simulink model "Simulink_disco"  (R2024a)
settings: Solver=VariableStepAuto  StartTime=0.0  StopTime=10.0  RelTol=1e-3
values from neighbouring files (symbols this model uses):
  k = 100    [Ec3.m]    (also in Simulink_datos.m)
  m = 10    [Ec3.m]    (also in Simulink_datos.m)
  r = 0.05    [Ec3.m]    (also in Simulink_datos.m)
settings Model: Creator=Braulio Ramíreza  LastModifiedBy=Braulio Ramíreza

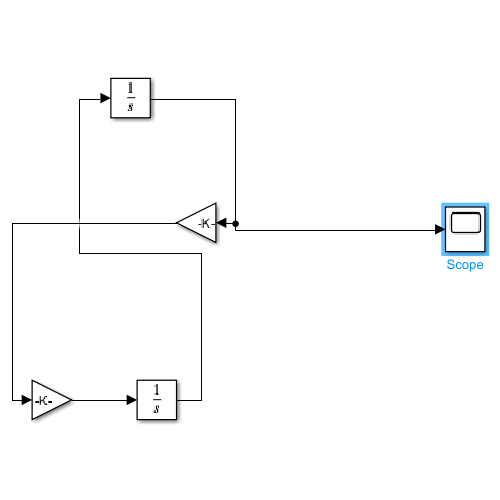
[thumbnail: Simulink's stored preview of the top-level diagram]
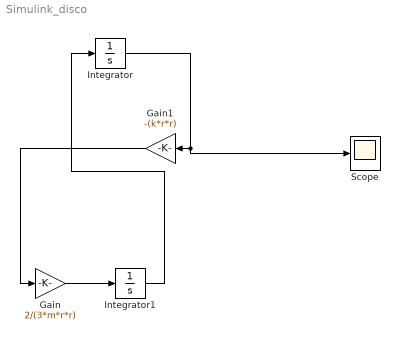
== system Simulink_disco ==
  Gain : Gain  Gain=2/(3*m*r*r)
  Gain1 : Gain  Gain=-(k*r*r)
  Integrator : Integrator
  Integrator1 : Integrator  InitialCondition=2
  Scope : Scope
  wires:
  Integrator1/1 -> Integrator/1
  Gain/1 -> Integrator1/1
  Gain1/1 -> Gain/1
  Integrator/1 -> Scope/1, Gain1/1
